simulink model "SimpleODE"  (Simulink 8.1)
settings: Solver=ode45  StartTime=0.0  StopTime=10.0  MaxStep=0.1  RelTol=1e-3
settings Model: Creator=gfaineko  LastModifiedBy=gfaineko
settings DataIOCC: LimitDataPoints=off  SignalLoggingSaveFormat=Dataset  DSMLogging=off
settings OptimizationCC: ExpressionDepthLimit=128
settings DebuggingCC: FcnCallInpInsideContextMsg=EnableAllAsError
settings GRTTargetCC: CombineOutputUpdateFcns=on  GRTInterface=off

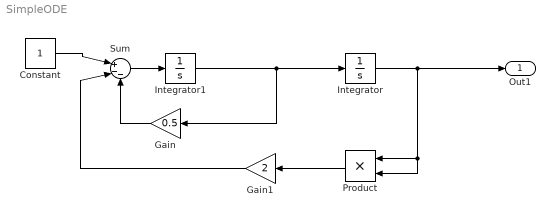
== system SimpleODE ==
  Constant : Constant
  Gain : Gain  Gain=0.5
  Gain1 : Gain  Gain=2
  Integrator : Integrator
  Integrator1 : Integrator
  Product : Product
  Sum : Sum  Inputs=|+--
  Out1 : Outport
  wires:
  Integrator/1 -> Product/2, Product/1, Out1/1
  Constant/1 -> Sum/1
  Sum/1 -> Integrator1/1
  Gain1/1 -> Sum/2
  Gain/1 -> Sum/3
  Integrator1/1 -> Gain/1, Integrator/1
  Product/1 -> Gain1/1
